simulink model "Mass_Spring_Damper_System"  (R2023b)
settings: Solver=VariableStepAuto  StartTime=0.0  StopTime=10.0  MaxStep=1e-3  RelTol=1e-3
undefined symbols (not defined in the file or in its folder): b, k, M, x0
settings Model: Creator=DELL  LastModifiedBy=DELL

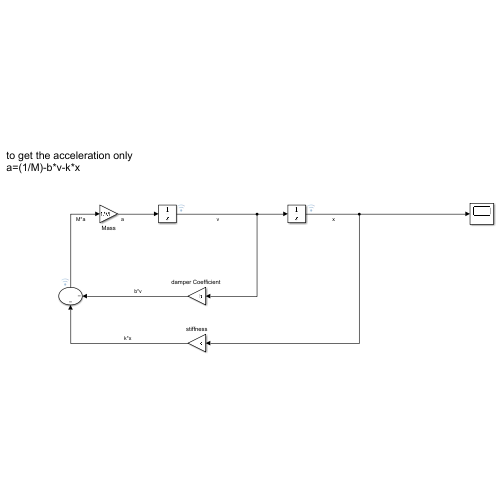
[thumbnail: Simulink's stored preview of the top-level diagram]
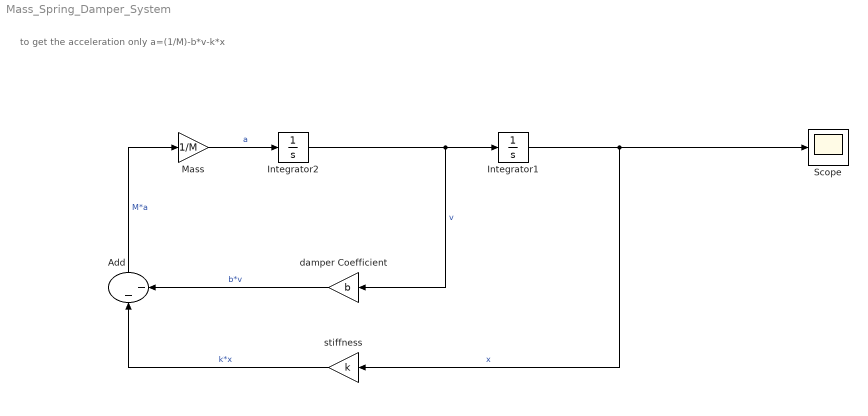
== system Mass_Spring_Damper_System ==
  note: to get the acceleration only
      | a=(1/M)-b*v-k*x
  Add : Sum  Inputs=|--
  Integrator1 : Integrator  InitialCondition=x0
  Integrator2 : Integrator
  Mass : Gain  Gain=1/M
  Scope : Scope
  "damper Coefficient " : Gain  Gain=b
  stiffness : Gain  Gain=k
  wires:
  Integrator2/1 -> "damper Coefficient "/1, Integrator1/1  "v"
  Integrator1/1 -> stiffness/1, Scope/1  "x"
  "damper Coefficient "/1 -> Add/2  "b*v"
  stiffness/1 -> Add/1  "k*x"
  Mass/1 -> Integrator2/1  "a"
  Add/1 -> Mass/1  "M*a"
